simulink model "short_line_transmission"  (Simulink 7.2)
settings: Solver=ode23t  StartTime=0.0  StopTime=0.1  RelTol=1e-6
libraries: powerlib x12, powerlib_extras x3, srolib x3
settings Model: Creator=user  LastModifiedBy=user

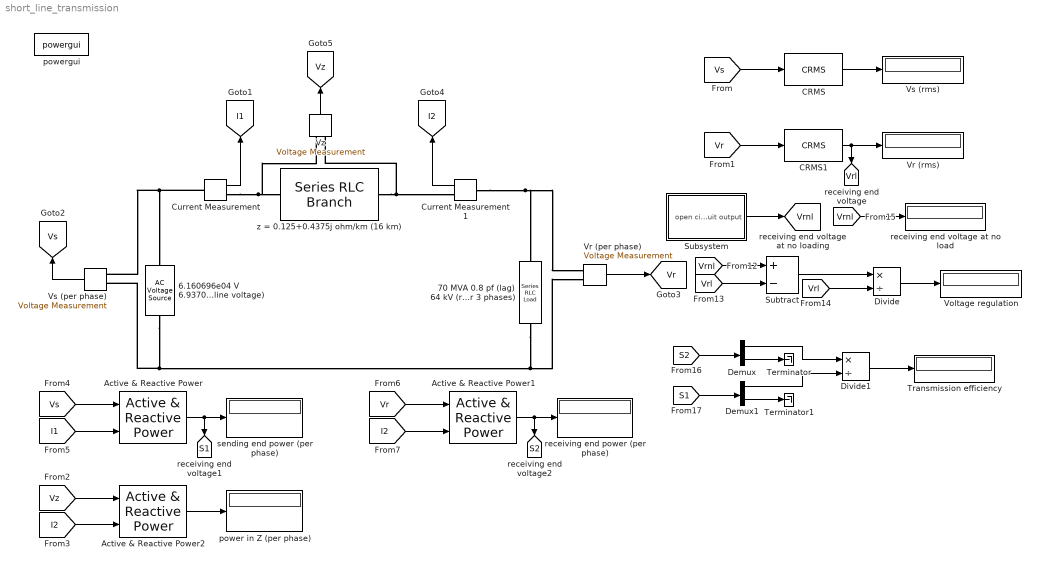
== system short_line_transmission ==
  6.160696e04 V 6.937054 deg (line voltage) : powerlib/Electrical Sources/AC Voltage Source  Orientation=up  DialogController=POWERSYS.PowerSysDialog  SystemSampleTime=-1  Amplitude=(3.556984e04)*1.414  Phase=6.937054  Frequency=60  SampleTime=-1  Measurements=Voltage
  70 MVA 0.8 pf (lag) 64 kV (rms) (for 3 phases) : powerlib/Elements/Series RLC Load  Orientation=down  DialogController=POWERSYS.PowerSysDialog  PhysicalDomain=powersysdomain  SubClassName=unknown  LeftPortType=p1  RightPortType=p1  LConnTagsString=a  RConnTagsString=__new0  NominalVoltage=64000/1.732  NominalFrequency=60  ActivePower=(70e6)*0.8/3  InductivePower=(70e6)*0.6/3  CapacitivePower=0  Setx0=off  InitialVoltage=0  SetiL0=off  InitialCurrent=0  Measurements=Branch voltage and current
  Active & Reactive Power : powerlib_extras/Measurements/Active & Reactive Power  DialogController=POWERSYS.PowerSysDialog  SystemSampleTime=-1  f1=60
  Active & Reactive Power1 : powerlib_extras/Measurements/Active & Reactive Power  DialogController=POWERSYS.PowerSysDialog  SystemSampleTime=-1  f1=60
  Active & Reactive Power2 : powerlib_extras/Measurements/Active & Reactive Power  DialogController=POWERSYS.PowerSysDialog  SystemSampleTime=-1  f1=60
  CRMS : srolib/RMS Blocks/CRMS  SystemSampleTime=-1
  CRMS1 : srolib/RMS Blocks/CRMS  SystemSampleTime=-1
  Current Measurement : powerlib/Measurements/Current Measurement  DialogController=POWERSYS.PowerSysDialog  SystemSampleTime=-1  PhasorSimulation=off  OutputType=Complex  PSBequivalent=0
  Current Measurement1 : powerlib/Measurements/Current Measurement  Orientation=left  DialogController=POWERSYS.PowerSysDialog  SystemSampleTime=-1  PhasorSimulation=off  OutputType=Complex  PSBequivalent=0
  Demux : Demux  Outputs=2
  Demux1 : Demux  Outputs=2
  Divide : Product  Inputs=*/  OutDataType=sfix(16)  OutScaling=2^-10
  Divide1 : Product  Inputs=*/  OutDataType=sfix(16)  OutScaling=2^-10
  Subsystem : Subsystem
  Subtract : Sum  Inputs=+-  OutDataType=sfix(16)  OutScaling=2^-10
  Terminator : Terminator
  Terminator1 : Terminator
  Transmission efficiency : Display
  Voltage regulation : Display
  Vr (per phase) : powerlib/Measurements/Voltage Measurement  DialogController=POWERSYS.PowerSysDialog  SystemSampleTime=-1  PhasorSimulation=off  OutputType=Complex  PSBequivalent=0
  Vr (rms) : Display
  Vs (per phase) : powerlib/Measurements/Voltage Measurement  Orientation=left  DialogController=POWERSYS.PowerSysDialog  SystemSampleTime=-1  PhasorSimulation=off  OutputType=Complex  PSBequivalent=0
  Vs (rms) : Display
  Vz : powerlib/Measurements/Voltage Measurement  Orientation=up  DialogController=POWERSYS.PowerSysDialog  SystemSampleTime=-1  PhasorSimulation=off  OutputType=Complex  PSBequivalent=0
  power in Z (per phase) : Display
  powergui : powerlib/powergui  SystemSampleTime=-1  SimulationMode=Continuous  SampleTime=50e-6  frequency=60  SPID=off  DisableSnubberDevices=off  DisableRonSwitches=off  DisableVfSwitches=off  SwTol=0  Interpol=off  frequencyindice=60  echomessages=off  HookPort=off  FunctionMessages=off  EnableUseOfTLC=off  x0status=blocks  RestoreLinks=warning  Frange=[0:2:500]  Ylog=off  Xlog=on  ShowGrid=off  save=off  variable=ZData  ZoomFFT=on  StartTime=0.0  cycles=1  DisplayStyle=1  fundamental=60  FreqAxis=off  MaxFrequency=1000  frequencyindicesteady=1  RmsSteady=1  display=off  Ts=0  methode=off
  receiving end power (per phase) : Display
  receiving end voltage at no load : Display
  sending end power (per phase) : Display
  z = 0.125+0.4375j ohm/km (16 km) : powerlib/Elements/Series RLC Branch  DialogController=POWERSYS.PowerSysDialog  PhysicalDomain=powersysdomain  SubClassName=unknown  LeftPortType=p1  RightPortType=p1  LConnTagsString=__new0  RConnTagsString=__new0  BranchType=RL  Resistance=0.125*16  Inductance=(0.4375/(120*3.14))*16  SetiL0=off  InitialCurrent=0  Capacitance=1e-6  Setx0=off  InitialVoltage=0  Measurements=Branch voltage and current
  tag scope: I1=global, I2=global, S1=global, S2=global, Vr=global, Vrl=global, Vrnl=global, Vs=global, Vz=global
  wires:
  Vr (per phase)/1 -> [Vr]
  Vs (per phase)/1 -> [Vs]
  [Vs] -> CRMS/1
  CRMS/1 -> Vs (rms)/1
  [Vr] -> CRMS1/1
  CRMS1/1 -> Vr (rms)/1, [Vrl]
  Active & Reactive Power/1 -> sending end power (per phase)/1, [S1]
  [Vs] -> Active & Reactive Power/1
  [I1] -> Active & Reactive Power/2
  Active & Reactive Power1/1 -> receiving end power (per phase)/1, [S2]
  [Vr] -> Active & Reactive Power1/1
  [I2] -> Active & Reactive Power1/2
  Active & Reactive Power2/1 -> power in Z (per phase)/1
  [Vz] -> Active & Reactive Power2/1
  [I2] -> Active & Reactive Power2/2
  Subsystem/1(open circuit output) -> [Vrnl]
  [Vrnl] -> Subtract/1
  Subtract/1 -> Divide/1
  Divide/1 -> Voltage regulation/1
  [Vrl] -> Subtract/2
  [Vrl] -> Divide/2
  [Vrnl] -> receiving end voltage at no load/1
  [S2] -> Demux/1
  Demux/2 -> Terminator/1
  [S1] -> Demux1/1
  Demux1/2 -> Terminator1/1
  Demux/1 -> Divide1/1
  Demux1/1 -> Divide1/2
  Divide1/1 -> Transmission efficiency/1
  Vz/1 -> [Vz]
  Current Measurement/1 -> [I1]
  Current Measurement1/1 -> [I2]
  connections:
  6.160696e04 V 6.937054 deg (line voltage)/LConn1 -- Vs (per phase)/LConn2 -- 70 MVA 0.8 pf (lag) 64 kV (rms) (for 3 phases)/RConn1 -- Vr (per phase)/LConn2
  z = 0.125+0.4375j ohm/km (16 km)/RConn1 -- Current Measurement1/RConn1 -- Vz/LConn2
  Current Measurement1/LConn1 -- 70 MVA 0.8 pf (lag) 64 kV (rms) (for 3 phases)/LConn1 -- Vr (per phase)/LConn1
  Current Measurement/RConn1 -- z = 0.125+0.4375j ohm/km (16 km)/LConn1 -- Vz/LConn1
  Current Measurement/LConn1 -- 6.160696e04 V 6.937054 deg (line voltage)/RConn1 -- Vs (per phase)/LConn1

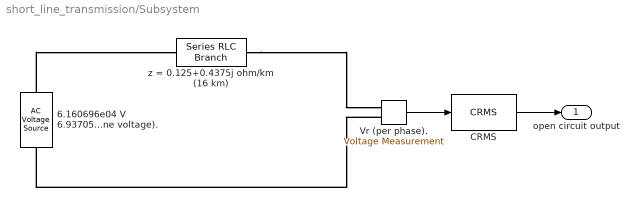
== system short_line_transmission/Subsystem ==
  6.160696e04 V 6.937054 deg (line voltage). : powerlib/Electrical Sources/AC Voltage Source  Orientation=up  DialogController=POWERSYS.PowerSysDialog  SystemSampleTime=-1  Amplitude=(3.556984e4)*1.414  Phase=6.937054  Frequency=60  SampleTime=-1  Measurements=Voltage
  CRMS : srolib/RMS Blocks/CRMS  SystemSampleTime=-1
  Vr (per phase). : powerlib/Measurements/Voltage Measurement  DialogController=POWERSYS.PowerSysDialog  SystemSampleTime=-1  PhasorSimulation=off  OutputType=Complex  PSBequivalent=0
  z = 0.125+0.4375j ohm/km (16 km) : powerlib/Elements/Series RLC Branch  DialogController=POWERSYS.PowerSysDialog  PhysicalDomain=powersysdomain  SubClassName=unknown  LeftPortType=p1  RightPortType=p1  LConnTagsString=__new0  RConnTagsString=__new0  BranchType=RL  Resistance=(0.125)*(16)  Inductance=(0.4375/(120*3.14))*(16)  SetiL0=off  InitialCurrent=0  Capacitance=1e-6  Setx0=off  InitialVoltage=0  Measurements=Branch voltage and current
  open circuit output : Outport
  wires:
  Vr (per phase)./1 -> CRMS/1
  CRMS/1 -> open circuit output/1
  connections:
  Vr (per phase)./LConn2 -- 6.160696e04 V 6.937054 deg (line voltage)./LConn1
  6.160696e04 V 6.937054 deg (line voltage)./RConn1 -- z = 0.125+0.4375j ohm/km (16 km)/LConn1
  z = 0.125+0.4375j ohm/km (16 km)/RConn1 -- Vr (per phase)./LConn1
